simulink library "HEV_Vehicle_Dynamics_Lib_org"  (Simulink 10.0)
settings: Solver=ode45  StartTime=0.0  StopTime=10.0  RelTol=1e-3  EnableMultiTasking=on
undefined symbols (not defined in the file): HEV_Param
libraries: fl_lib x22, nesl_utility x11, fl_ps_legacy_lib x10, sdl_lib x4, $bdroot x1
Description:
  | Copyright 2014-2017 The MathWorks, Inc.
settings Model: Creator=smiller  LastModifiedBy=bhisma

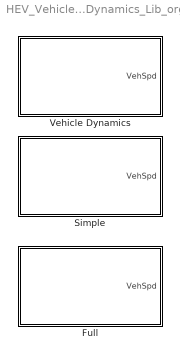
== system HEV_Vehicle_Dynamics_Lib_org ==
  Full : Subsystem
      mask Display:
      | image(imread('HEV_Vehicle_Dynamics_Full_IMAGE.jpg'));
      | port_label('LConn',1,'Sh');
      | port_label('output',1,'Spd');
  Simple : Subsystem  mask(Rigid vehicle model){mass=HEV_Param.Vehicle.Mass, area=HEV_Param.Vehicle.Frontal_Area, Cd=HEV_Param.Vehicle.Aero_Drag_Coeff, radius=HEV_Param.Vehicle.Tire_Radius, wheel_inertia=HEV_Param.Vehicle.Wheel_Inertia, gear_ratio=HEV_Param.Vehicle.Engine_Vehicle_Gear_Ratio}
      mask prompts: mass "Mass (Kg)"; area "Frontal Area (m^2)"; Cd "Drag coefficient"; radius "Tire radius (m)"; wheel_inertia "Total wheel inertia (kg*m^2)"; gear_ratio "Engine to vehicle gear ratio"
      mask help: Model vehicle effective inertia and drag force as seen by the engine. It is assumed that the vehicle is moving on flat terrain. No bearing friction or gear losses are included.
      mask init:
      | gravity = 9.81;
      mask Display:
      | image(imread('HEV_Vehicle_Dynamics_Simple_IMAGE.jpg'));
      | port_label('LConn',1,'Sh');
      | port_label('output',1,'Spd');
  Vehicle Dynamics : Subsystem  BlockChoice=Simple
      settings: TemplateBlock=self  MemberBlocks=Full,Simple
      mask Display:
      | port_label('LConn',1,'Sh');
      | port_label('output',1,'Spd');

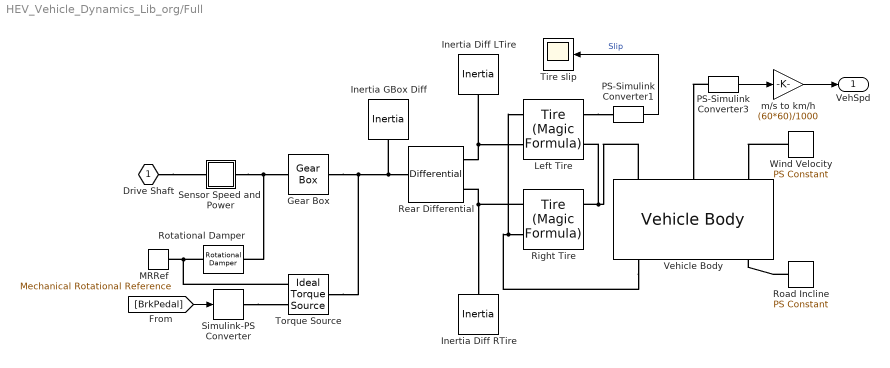
== system HEV_Vehicle_Dynamics_Lib_org/Full ==
  Gear Box : fl_lib/Mechanical/Mechanisms/Gear Box  ratio=HEV_Param.Vehicle.Engine_Vehicle_Gear_Ratio  t_in_specify=off  t_in_priority=High  t_in=0 N*m  t_in_nominal_specify=off  t_in_nominal_unit=N*m  t_in_nominal_value=1  t_out_specify=off  t_out_priority=High  t_out=0 N*m  t_out_nominal_specify=off  t_out_nominal_unit=N*m  t_out_nominal_value=1
  Inertia Diff LTire : fl_lib/Mechanical/Rotational Elements/Inertia  inertia=HEV_Param.Vehicle.Wheel_Inertia*2 kg*m^2  w_specify=on  w_priority=High  w=0 rad/s  w_nominal_specify=off  w_nominal_unit=rad/s  w_nominal_value=1  t_specify=off  t_priority=High  t=0 N*m  t_nominal_specify=off  t_nominal_unit=N*m  t_nominal_value=1
  Inertia Diff RTire : fl_lib/Mechanical/Rotational Elements/Inertia  inertia=HEV_Param.Vehicle.Wheel_Inertia*2 kg*m^2  w_specify=on  w_priority=High  w=0 rad/s  w_nominal_specify=off  w_nominal_unit=rad/s  w_nominal_value=1  t_specify=off  t_priority=High  t=0 N*m  t_nominal_specify=off  t_nominal_unit=N*m  t_nominal_value=1
  Inertia GBox Diff : fl_lib/Mechanical/Rotational Elements/Inertia  inertia=HEV_Param.Vehicle.Trans.Inertia kg*m^2  w_specify=on  w_priority=High  w=0 rad/s  w_nominal_specify=off  w_nominal_unit=rad/s  w_nominal_value=1  t_specify=off  t_priority=High  t=0 N*m  t_nominal_specify=off  t_nominal_unit=N*m  t_nominal_value=1
  Left Tire : sdl_lib/Tires & Vehicles/Tire (Magic Formula)  parameterization=1  F_z1=HEV_Param.Vehicle.Tire.Rated_Vertical_Load N  F_x1=HEV_Param.Vehicle.Tire.Rated_Peak_Long_Force N  kappa1=HEV_Param.Vehicle.Tire.Slip_At_Peak_Force  B_m=10  C_m=1.9  D_m=1  E_m=0.97  fz0=4e+3 N  p_Cx=1.685  p_Dx=[ 1.21 -0.037 ]  p_Ex=[ 0.344 0.095 -0.02 0 ]  p_Kx=[ 21.51 -0.163 0.245 ]  p_Hx=[ -0.002 0.002 ]  p_Vx=[ 0 0 ]  v_tr_thr=0.1 m/s  r_e=HEV_Param.Vehicle.Tire_Radius m  model_compliance=0  stiffness=1e+6 N/m  damping=1000 N/(m/s)  model_inertia=1  inertia=1e-2 kg*m^2  initial_velocity=0 rpm  model_resistance=0  resistance_model=1  coeff=0.015  p_tire=250e3 Pa  alpha=-0.003  beta=0.97  coeff_a=84e-4  coeff_b=6.2e-4 s/m  coeff_c=1.6e-4 s^2/m^2  v_thr=1e-3 m/s
      settings: SourceProductName=Simscape Driveline
  MRRef : fl_lib/Mechanical/Rotational Elements/Mechanical Rotational Reference
  PS-Simulink Converter1 : nesl_utility/PS-Simulink Converter  PhysicalDomain=network_engine_domain  SubClassName=ps_output  LeftPortType=input  RightPortType=output  PseudoPeriodic=off  Frequencies=[]  Unit=1  AffineConversion=off
  PS-Simulink Converter3 : nesl_utility/PS-Simulink Converter  PhysicalDomain=network_engine_domain  SubClassName=ps_output  LeftPortType=input  RightPortType=output  PseudoPeriodic=off  Frequencies=[]  Unit=m/s  AffineConversion=off
  Rear Differential : sdl_lib/Gears/Differential  driveshaft_location=2  cd_ratio=1  friction_model=1  efficiency=[ 0.85 0.92 ]  mu_visc=[ 0 0 ] N*m/(rad/s)  pwr_thr=[ 0.001 0.001 ] W  carrier_inertia=0 kg*m^2  planet_inertia=0 kg*m^2  temperature_TLU=[ 280 300 320 ] K  efficiency_ss_TLU=[ 0.95 0.9 0.85 ]  efficiency_cd_TLU=[ 0.95 0.9 0.85 ]  thermal_mass=50 J/K  T_init=300 K
      settings: SourceProductName=Simscape Driveline  SourceProductBaseCode=LD
  Right Tire : sdl_lib/Tires & Vehicles/Tire (Magic Formula)  parameterization=1  F_z1=HEV_Param.Vehicle.Tire.Rated_Vertical_Load N  F_x1=HEV_Param.Vehicle.Tire.Rated_Peak_Long_Force N  kappa1=HEV_Param.Vehicle.Tire.Slip_At_Peak_Force  B_m=10  C_m=1.9  D_m=1  E_m=0.97  fz0=4e+3 N  p_Cx=1.685  p_Dx=[ 1.21 -0.037 ]  p_Ex=[ 0.344 0.095 -0.02 0 ]  p_Kx=[ 21.51 -0.163 0.245 ]  p_Hx=[ -0.002 0.002 ]  p_Vx=[ 0 0 ]  v_tr_thr=0.1 m/s  r_e=HEV_Param.Vehicle.Tire_Radius m  model_compliance=0  stiffness=1e+6 N/m  damping=1000 N/(m/s)  model_inertia=1  inertia=1e-2 kg*m^2  initial_velocity=0 rpm  model_resistance=0  resistance_model=1  coeff=0.015  p_tire=250e3 Pa  alpha=-0.003  beta=0.97  coeff_a=84e-4  coeff_b=6.2e-4 s/m  coeff_c=1.6e-4 s^2/m^2  v_thr=1e-3 m/s
      settings: SourceProductName=Simscape Driveline
  Road Incline : fl_lib/Physical Signals/Sources/PS Constant  constant=HEV_Param.Vehicle.Incline
  Rotational Damper : fl_lib/Mechanical/Rotational Elements/Rotational Damper  D=HEV_Param.Vehicle.Trans.Friction N*m/(rad/s)  w_specify=off  w_priority=High  w=0 rad/s  w_nominal_specify=off  w_nominal_unit=rad/s  w_nominal_value=1  t_specify=off  t_priority=High  t=0 N*m  t_nominal_specify=off  t_nominal_unit=N*m  t_nominal_value=1
  Sensor Speed and  Power : Subsystem
      mask Display: disp('S')
  Simulink-PS Converter : nesl_utility/Simulink-PS Converter  PhysicalDomain=network_engine_domain  SubClassName=ps_input  LeftPortType=input  RightPortType=output  PseudoPeriodic=off  Frequencies=[]  NoiseDistribution=none  NoiseParameters=[]  Unit=1  AffineConversion=off  FilteringAndDerivatives=zero  SimscapeFilterOrder=1  InputFilterTimeConstant=0.001  UdotUserProvided=1
  Tire slip : Scope
  Torque Source : fl_lib/Mechanical/Mechanical Sources/Ideal Torque Source
  Vehicle Body : sdl_lib/Tires & Vehicles/Vehicle Body  mass=HEV_Param.Vehicle.Mass kg  n_w=2  x_f=HEV_Param.Vehicle.Distance_CG_FrontAxle m  x_r=HEV_Param.Vehicle.Distance_CG_RearAxle m  y_c=HEV_Param.Vehicle.Distance_CG_Ground m  mass_var=simscape.enum.onoff.off  model_pitch=simscape.enum.onoff.off  inertia=4000 kg*m^2  suspension_model=sdl.enum.linearTLU.linear  k_f=1e4 N/m  b_f=1e4 N/(m/s)  k_r=1e4 N/m  b_r=1e4 N/(m/s)  k_f_TLU=[-2000, -1000, 0, 1000, 2000] N  x_f_TLU=[-.4, -.2, 0, .2, .4] m  b_f_TLU=[-200, -100, 0, 100, 200] N  v_f_TLU=[-4, -2, 0, 2, 4] m/s  k_r_TLU=[-2000, -1000, 0, 1000, 2000] N  x_r_TLU=[-.4, -.2, 0, .2, .4] m  b_r_TLU=[-200, -100, 0, 100, 200] N  v_r_TLU=[-4, -2, 0, 2, 4] m/s  interp_method=simscape.enum.interpolation.linear  extrap_method=simscape.enum.extrapolation.linear  model_hardstop=simscape.enum.onoff.off  upper_bound_f=.25 m  lower_bound_f=-.25 m  stop_k_f=1e6 N/m  stop_b_f=150 N/(m/s)  upper_bound_r=.25 m  lower_bound_r=-.25 m  stop_k_r=1e6 N/m  stop_b_r=150 N/(m/s)  initial_pitch=0 rad  initial_pitch_rate=0 rad/s  g=9.81 m/s^2  liftoff_warning=simscape.enum.onoff.off  area=HEV_Param.Vehicle.Frontal_Area m^2  Cd=HEV_Param.Vehicle.Aero_Drag_Coeff  rho=1.18 kg/m^3  v_specify=on  v_priority=High  v=0 m/s  v_nominal_specify=off  v_nominal_unit=m/s  v_nominal_value=1
      settings: SourceProductName=Simscape Driveline
  Wind Velocity : fl_lib/Physical Signals/Sources/PS Constant  constant=0
  m/s to km/h : Gain  Gain=(60*60)/1000
  Drive Shaft : PMIOPort  Side=Left
  VehSpd : Outport
  wires:
  PS-Simulink Converter3/1 -> m/s to km/h/1
  m/s to km/h/1 -> VehSpd/1
  PS-Simulink Converter1/1 -> Tire slip/1  "Slip"
  [BrkPedal] -> Simulink-PS Converter/1
  connections:
  Right Tire/RConn2 -- Vehicle Body/LConn1 -- Left Tire/RConn2
  Right Tire/LConn1 -- Vehicle Body/RConn1 -- Left Tire/LConn1
  Road Incline/RConn1 -- Vehicle Body/RConn3
  Wind Velocity/RConn1 -- Vehicle Body/LConn3
  PS-Simulink Converter3/LConn1 -- Vehicle Body/LConn2
  Left Tire/RConn1 -- PS-Simulink Converter1/LConn1
  Rear Differential/RConn2 -- Left Tire/LConn2 -- Inertia Diff LTire/LConn1
  Right Tire/LConn2 -- Rear Differential/RConn1 -- Inertia Diff RTire/LConn1
  Gear Box/RConn1 -- Torque Source/LConn1 -- Rear Differential/LConn1 -- Inertia GBox Diff/LConn1
  Sensor Speed and  Power/RConn1 -- Gear Box/LConn1 -- Rotational Damper/LConn1
  Rotational Damper/RConn1 -- Torque Source/RConn2 -- MRRef/LConn1
  Drive Shaft/RConn1 -- Sensor Speed and  Power/LConn1
  Simulink-PS Converter/RConn1 -- Torque Source/RConn1

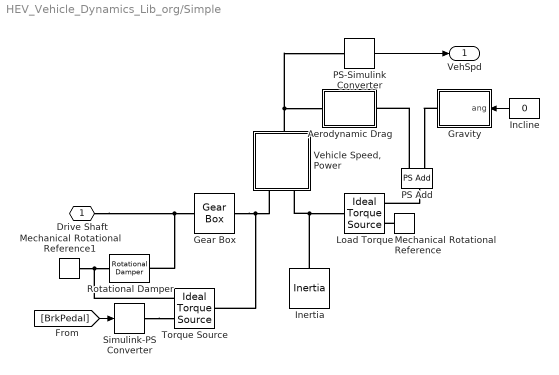
== system HEV_Vehicle_Dynamics_Lib_org/Simple ==
  Aerodynamic Drag : Subsystem
  Gear Box : fl_lib/Mechanical/Mechanisms/Gear Box  ratio=gear_ratio  t_in_specify=off  t_in_priority=High  t_in=0 N*m  t_in_nominal_specify=off  t_in_nominal_unit=N*m  t_in_nominal_value=1  t_out_specify=off  t_out_priority=High  t_out=0 N*m  t_out_nominal_specify=off  t_out_nominal_unit=N*m  t_out_nominal_value=1
  Gravity : Subsystem
  Incline : Constant  Value=0
  Inertia : fl_lib/Mechanical/Rotational Elements/Inertia  inertia=mass*radius*radius kg*m^2  w_specify=off  w_priority=High  w=0 rad/s  w_nominal_specify=off  w_nominal_unit=rad/s  w_nominal_value=1  t_specify=off  t_priority=None  t=0 N*m  t_nominal_specify=off  t_nominal_unit=N*m  t_nominal_value=1
  Load Torque : fl_lib/Mechanical/Mechanical Sources/Ideal Torque Source
  Mechanical Rotational Reference : fl_lib/Mechanical/Rotational Elements/Mechanical Rotational Reference
  Mechanical Rotational Reference1 : fl_lib/Mechanical/Rotational Elements/Mechanical Rotational Reference
  PS Add : fl_ps_legacy_lib/Legacy Physical Signals/Functions/PS Add
      settings: SourceProductName=Simscape  SourceProductBaseCode=SS  InternalSimscapePortConfiguration="{\"Bottom\":[],\"Left\":[{\"id\":\"I1\",\"label\":\"\",\"type\":\"input\"},{\"id\":\"I2\",\"label\":\"\",\"type\":\"input\"}],\"Right\":[{\"id\":\"O\",\"label\":\"\",\"type\":\"output\"}],\"Top\":[]}"
  PS-Simulink Converter : nesl_utility/PS-Simulink Converter  PhysicalDomain=network_engine_domain  SubClassName=ps_output  LeftPortType=input  RightPortType=output  PseudoPeriodic=off  Frequencies=[]  Unit=1  AffineConversion=off
  Rotational Damper : fl_lib/Mechanical/Rotational Elements/Rotational Damper  D=HEV_Param.Vehicle.Trans.Friction N*m/(rad/s)  w_specify=off  w_priority=High  w=0 rad/s  w_nominal_specify=off  w_nominal_unit=rad/s  w_nominal_value=1  t_specify=off  t_priority=High  t=0 N*m  t_nominal_specify=off  t_nominal_unit=N*m  t_nominal_value=1
  Simulink-PS Converter : nesl_utility/Simulink-PS Converter  PhysicalDomain=network_engine_domain  SubClassName=ps_input  LeftPortType=input  RightPortType=output  PseudoPeriodic=off  Frequencies=[]  NoiseDistribution=none  NoiseParameters=[]  Unit=1  AffineConversion=off  FilteringAndDerivatives=zero  SimscapeFilterOrder=1  InputFilterTimeConstant=0.001  UdotUserProvided=1
  Torque Source : fl_lib/Mechanical/Mechanical Sources/Ideal Torque Source
  "Vehicle Speed, Power" : Subsystem
  Drive Shaft : PMIOPort  Side=Left
  VehSpd : Outport
  wires:
  PS-Simulink Converter/1 -> VehSpd/1
  [BrkPedal] -> Simulink-PS Converter/1
  Incline/1 -> Gravity/1(ang)
  connections:
  Rotational Damper/LConn1 -- Drive Shaft/RConn1 -- Gear Box/LConn1
  "Vehicle Speed, Power"/RConn1 -- PS-Simulink Converter/LConn1 -- Aerodynamic Drag/LConn1
  PS Add/LConn2 -- Aerodynamic Drag/RConn1
  Mechanical Rotational Reference/LConn1 -- Load Torque/RConn2
  Inertia/LConn1 -- Load Torque/LConn1 -- "Vehicle Speed, Power"/LConn2
  Mechanical Rotational Reference1/LConn1 -- Torque Source/RConn2 -- Rotational Damper/RConn1
  Gear Box/RConn1 -- Torque Source/LConn1 -- "Vehicle Speed, Power"/LConn1
  Simulink-PS Converter/RConn1 -- Torque Source/RConn1
  PS Add/RConn1 -- Load Torque/RConn1
  Gravity/RConn1 -- PS Add/LConn1

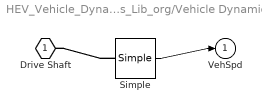
== system HEV_Vehicle_Dynamics_Lib_org/Vehicle Dynamics ==
  Simple : $bdroot/Simple  mass=HEV_Param.Vehicle.Mass  area=HEV_Param.Vehicle.Frontal_Area  Cd=HEV_Param.Vehicle.Aero_Drag_Coeff  radius=HEV_Param.Vehicle.Tire_Radius  wheel_inertia=HEV_Param.Vehicle.Wheel_Inertia  gear_ratio=HEV_Param.Vehicle.Engine_Vehicle_Gear_Ratio
  Drive Shaft : PMIOPort  Side=Left
  VehSpd : Outport
  wires:
  Simple/1 -> VehSpd/1
  connections:
  Simple/LConn1 -- Drive Shaft/RConn1

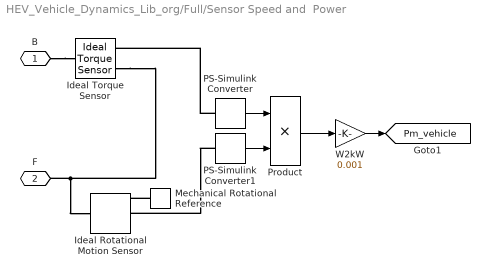
== system HEV_Vehicle_Dynamics_Lib_org/Full/Sensor Speed and  Power ==
  Ideal Rotational Motion Sensor : fl_lib/Mechanical/Mechanical Sensors/Ideal Rotational Motion Sensor  offset=0 rad
  Ideal Torque Sensor : fl_lib/Mechanical/Mechanical Sensors/Ideal Torque Sensor
  Mechanical Rotational Reference : fl_lib/Mechanical/Rotational Elements/Mechanical Rotational Reference
  PS-Simulink Converter : nesl_utility/PS-Simulink Converter  PhysicalDomain=network_engine_domain  SubClassName=ps_output  LeftPortType=input  RightPortType=output  PseudoPeriodic=off  Frequencies=[]  Unit=N*m  AffineConversion=off
  PS-Simulink Converter1 : nesl_utility/PS-Simulink Converter  PhysicalDomain=network_engine_domain  SubClassName=ps_output  LeftPortType=input  RightPortType=output  PseudoPeriodic=off  Frequencies=[]  Unit=rad/s  AffineConversion=off
  Product : Product  RndMeth=Zero
  W2kW : Gain  Gain=0.001
  B : PMIOPort  Side=Left
  F : PMIOPort  Port=2  Side=Right
  tag scope: Pm_vehicle=global
  wires:
  PS-Simulink Converter1/1 -> Product/2
  PS-Simulink Converter/1 -> Product/1
  Product/1 -> W2kW/1
  W2kW/1 -> [Pm_vehicle]
  connections:
  PS-Simulink Converter1/LConn1 -- Ideal Rotational Motion Sensor/RConn2
  PS-Simulink Converter/LConn1 -- Ideal Torque Sensor/RConn2
  B/RConn1 -- Ideal Torque Sensor/LConn1
  Ideal Torque Sensor/RConn1 -- F/RConn1 -- Ideal Rotational Motion Sensor/LConn1
  Mechanical Rotational Reference/LConn1 -- Ideal Rotational Motion Sensor/RConn1

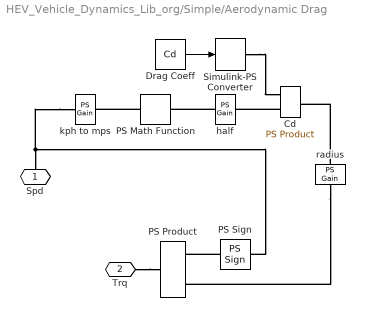
== system HEV_Vehicle_Dynamics_Lib_org/Simple/Aerodynamic Drag ==
  Cd : fl_ps_legacy_lib/Legacy Physical Signals/Functions/PS Product
      settings: SourceProductName=Simscape  SourceProductBaseCode=SS
  Drag Coeff : Constant  Value=Cd
  PS Math Function : fl_ps_legacy_lib/Legacy Physical Signals/Functions/PS Math Function  fcn_choice=7
      settings: SourceProductName=Simscape  SourceProductBaseCode=SS  InternalSimscapePortConfiguration="{\"Bottom\":[],\"Left\":[{\"id\":\"I\",\"label\":\"\",\"type\":\"input\"}],\"Right\":[{\"id\":\"O\",\"label\":\"\",\"type\":\"output\"}],\"Top\":[]}"
  PS Product : fl_ps_legacy_lib/Legacy Physical Signals/Functions/PS Product
      settings: SourceProductName=Simscape  SourceProductBaseCode=SS
  PS Sign : fl_ps_legacy_lib/Legacy Physical Signals/Nonlinear Operators/PS Sign
      settings: SourceProductName=Simscape  SourceProductBaseCode=SS  InternalSimscapePortConfiguration="{\"Bottom\":[],\"Left\":[{\"id\":\"I\",\"label\":\"\",\"type\":\"input\"}],\"Right\":[{\"id\":\"O\",\"label\":\"\",\"type\":\"output\"}],\"Top\":[]}"
  Simulink-PS Converter : nesl_utility/Simulink-PS Converter  PhysicalDomain=network_engine_domain  SubClassName=ps_input  LeftPortType=input  RightPortType=output  PseudoPeriodic=off  Frequencies=[]  NoiseDistribution=none  NoiseParameters=[]  Unit=1  AffineConversion=off  FilteringAndDerivatives=zero  SimscapeFilterOrder=1  InputFilterTimeConstant=.001  UdotUserProvided=0
  half : fl_ps_legacy_lib/Legacy Physical Signals/Functions/PS Gain  gain=1/2
      settings: SourceProductName=Simscape
  kph to mps : fl_ps_legacy_lib/Legacy Physical Signals/Functions/PS Gain  gain=1/3.6
      settings: SourceProductName=Simscape
  radius : fl_ps_legacy_lib/Legacy Physical Signals/Functions/PS Gain  gain=-radius
      settings: SourceProductName=Simscape
  Spd : PMIOPort  Side=Left
  Trq : PMIOPort  Port=2  Side=Right
  wires:
  Drag Coeff/1 -> Simulink-PS Converter/1
  connections:
  Simulink-PS Converter/RConn1 -- Cd/LConn1
  PS Sign/RConn1 -- PS Product/LConn2
  radius/LConn1 -- Cd/RConn1
  radius/RConn1 -- PS Product/LConn1
  Cd/LConn2 -- half/RConn1
  PS Math Function/LConn1 -- kph to mps/RConn1
  half/LConn1 -- PS Math Function/RConn1
  kph to mps/LConn1 -- PS Sign/LConn1 -- Spd/RConn1
  Trq/RConn1 -- PS Product/RConn1

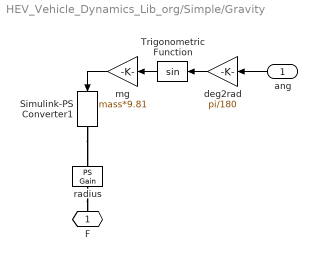
== system HEV_Vehicle_Dynamics_Lib_org/Simple/Gravity ==
  ang : Inport
  Simulink-PS Converter1 : nesl_utility/Simulink-PS Converter  PhysicalDomain=network_engine_domain  SubClassName=ps_input  LeftPortType=input  RightPortType=output  PseudoPeriodic=off  Frequencies=[]  NoiseDistribution=none  NoiseParameters=[]  Unit=1  AffineConversion=off  FilteringAndDerivatives=zero  SimscapeFilterOrder=1  InputFilterTimeConstant=0.001  UdotUserProvided=1
  Trigonometric Function : Trigonometry
  deg2rad : Gain  Gain=pi/180
  mg : Gain  Gain=mass*9.81
  radius : fl_ps_legacy_lib/Legacy Physical Signals/Functions/PS Gain  gain=-radius
      settings: SourceProductName=Simscape
  F : PMIOPort  Side=Right
  wires:
  mg/1 -> Simulink-PS Converter1/1
  deg2rad/1 -> Trigonometric Function/1
  ang/1 -> deg2rad/1
  Trigonometric Function/1 -> mg/1
  connections:
  Simulink-PS Converter1/RConn1 -- radius/LConn1
  radius/RConn1 -- F/RConn1

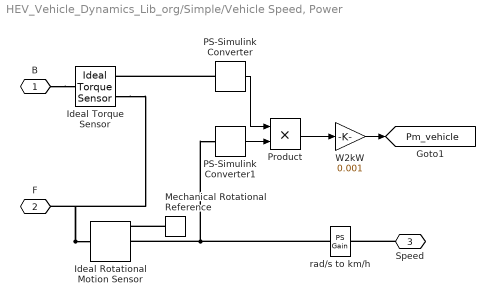
== system HEV_Vehicle_Dynamics_Lib_org/Simple/Vehicle Speed, Power ==
  Ideal Rotational Motion Sensor : fl_lib/Mechanical/Mechanical Sensors/Ideal Rotational Motion Sensor  offset=0 rad
  Ideal Torque Sensor : fl_lib/Mechanical/Mechanical Sensors/Ideal Torque Sensor
  Mechanical Rotational Reference : fl_lib/Mechanical/Rotational Elements/Mechanical Rotational Reference
  PS-Simulink Converter : nesl_utility/PS-Simulink Converter  PhysicalDomain=network_engine_domain  SubClassName=ps_output  LeftPortType=input  RightPortType=output  PseudoPeriodic=off  Frequencies=[]  Unit=N*m  AffineConversion=off
  PS-Simulink Converter1 : nesl_utility/PS-Simulink Converter  PhysicalDomain=network_engine_domain  SubClassName=ps_output  LeftPortType=input  RightPortType=output  PseudoPeriodic=off  Frequencies=[]  Unit=rad/s  AffineConversion=off
  Product : Product  RndMeth=Zero
  W2kW : Gain  Gain=0.001
  rad/s to km/h : fl_ps_legacy_lib/Legacy Physical Signals/Functions/PS Gain  gain=radius*3.6
      settings: SourceProductName=Simscape
  B : PMIOPort  Side=Left
  F : PMIOPort  Port=2  Side=Left
  Speed : PMIOPort  Port=3  Side=Right
  tag scope: Pm_vehicle=global
  wires:
  W2kW/1 -> [Pm_vehicle]
  Product/1 -> W2kW/1
  PS-Simulink Converter/1 -> Product/1
  PS-Simulink Converter1/1 -> Product/2
  connections:
  Mechanical Rotational Reference/LConn1 -- Ideal Rotational Motion Sensor/RConn1
  Ideal Rotational Motion Sensor/LConn1 -- F/RConn1 -- Ideal Torque Sensor/RConn1
  B/RConn1 -- Ideal Torque Sensor/LConn1
  PS-Simulink Converter/LConn1 -- Ideal Torque Sensor/RConn2
  rad/s to km/h/LConn1 -- Ideal Rotational Motion Sensor/RConn2 -- PS-Simulink Converter1/LConn1
  Speed/RConn1 -- rad/s to km/h/RConn1
